simulink model "racing_car2_MPC"  (R2019b)
settings: Solver=ode3  StartTime=0.0  StopTime=203  FixedStep=1/60  MaxStep=1/60  MinStep=1/60  RelTol=1e-3  EnableMultiTasking=on
values from neighbouring files (symbols this model uses):
  params = load(param_file)    [initialize.m]    (also in old.mat = )
  reference = [0 2.199971 4.399665 6.599066 8.798417 10.997994 13.19795 15.398175 17.598331 19.798309 21.998281 24.198335 ... (12006 elements, 2001x6)]    [0410_night_94s.mat]    (also in data60-93.88.mat; initialize.m = data0; old.mat = [0 2.199956 4.399633 6.599016 8.798347 10.997905 13.197843 1)
settings Model: Creator=Administrator  LastModifiedBy=Catherine
settings DataIOCC: LimitDataPoints=on  SaveFormat=Array  ReturnWorkspaceOutputs=off
settings OptimizationCC: LifeSpan=inf
settings DebuggingCC: UnderspecifiedInitializationDetection=Classic  MergeDetectMultiDrivingBlocksExec=none  SolverPrmCheckMsg=warning  StateNameClashWarn=warning  SFUnexpectedBacktrackingDiag=warning  SFNoUnconditionalDefaultTransitionDiag=warning  SFExecutionAtInitializationDiag=none  ArithmeticOperatorsInVariantConditions=warning
settings HardwareCC: ProdBitPerPointer=32  ProdBitPerSizeT=32  ProdBitPerPtrDiffT=32  ProdLargestAtomicFloat=None  ProdIntDivRoundTo=Undefined  ProdEndianess=Unspecified  ProdWordSize=32  ProdHWDeviceType=32-bit Generic
settings ModelReferenceCC: PropagateSignalLabelsOutOfModel=off
settings SFSimCC: SimUseLocalCustomCode=off  CustomCodeUndefinedFunction=UseInterfaceOnly
settings RTWCC: RTWUseLocalCustomCode=off
settings CodeAppCC: StateflowObjectComments=on
settings GRTTargetCC: TargetLangStandard=C89/C90 (ANSI)  GeneratePreprocessorConditionals=Disable all
settings ConfigComp: CovMetricSettings=dw  CovHtmlReporting=on  CovSaveCumulativeToWorkspaceVar=on  CovSaveSingleToWorkspaceVar=on  CovExternalEMLEnable=off

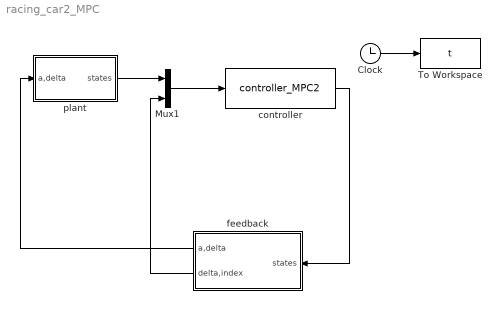
== system racing_car2_MPC ==
  Clock : Clock
  Mux1 : Mux  Inputs=2
  To Workspace : ToWorkspace  VariableName=t  SampleTime=-1
  controller : S-Function  FunctionName=controller_MPC2  Parameters=reference,params  SFunctionDeploymentMode=off  EnableBusSupport=off
  feedback : Subsystem
  plant : Subsystem
  wires:
  Mux1/1 -> controller/1
  plant/1(states) -> Mux1/1
  feedback/1(a,delta) -> plant/1(a,delta)
  Clock/1 -> To Workspace/1
  controller/1 -> feedback/1(states)
  feedback/2(delta,index) -> Mux1/2

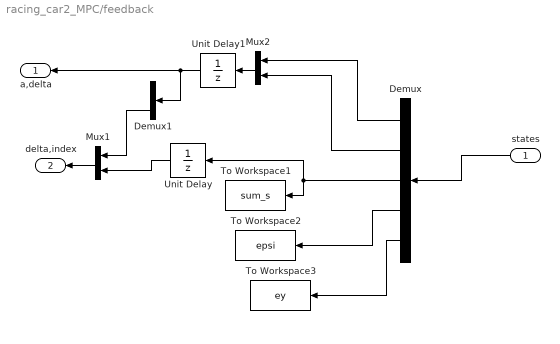
== system racing_car2_MPC/feedback ==
  states : Inport
  Demux : Demux  Outputs=5
  Demux1 : Demux  Outputs=2
  Mux1 : Mux  Inputs=2
  Mux2 : Mux  Inputs=2
  To Workspace1 : ToWorkspace  VariableName=sum_s  SampleTime=-1
  To Workspace2 : ToWorkspace  VariableName=epsi  SampleTime=-1
  To Workspace3 : ToWorkspace  VariableName=ey  SampleTime=-1
  Unit Delay : UnitDelay  SampleTime=-1  HasFrameUpgradeWarning=on
  Unit Delay1 : UnitDelay  SampleTime=-1  HasFrameUpgradeWarning=on
  a,delta : Outport
  delta,index : Outport  Port=2
  wires:
  states/1 -> Demux/1
  Demux/1 -> Mux2/1
  Demux/3 -> Unit Delay/1, To Workspace1/1
  Demux/4 -> To Workspace2/1
  Demux/5 -> To Workspace3/1
  Unit Delay1/1 -> Demux1/1, a,delta/1
  Mux2/1 -> Unit Delay1/1
  Demux/2 -> Mux2/2
  Unit Delay/1 -> Mux1/2
  Mux1/1 -> delta,index/1
  Demux1/2 -> Mux1/1

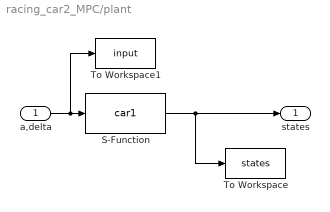
== system racing_car2_MPC/plant ==
  a,delta : Inport
  S-Function : S-Function  FunctionName=car1  Parameters=init  SFunctionDeploymentMode=off  EnableBusSupport=off
  To Workspace : ToWorkspace  VariableName=states  SampleTime=-1
  To Workspace1 : ToWorkspace  VariableName=input  SampleTime=-1
  states : Outport
  wires:
  a,delta/1 -> To Workspace1/1, S-Function/1
  S-Function/1 -> states/1, To Workspace/1
